simulink model "syste_analysis_i"  (R2024a)
settings: Solver=FixedStepAuto  StartTime=0.0  StopTime=10  FixedStep=0.01  RelTol=1e-3
undefined symbols (not defined in the file or in its folder): A_stable, B_num
settings Model: Creator=phili  LastModifiedBy=phili

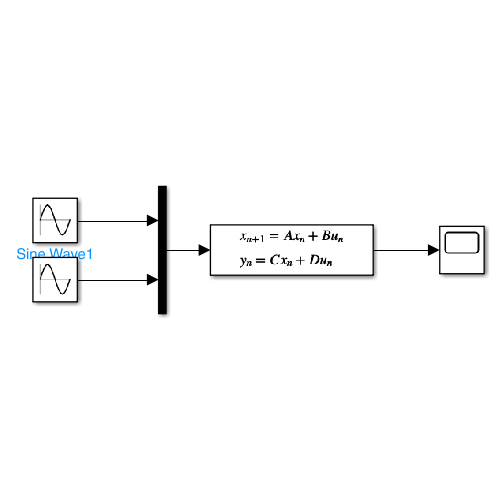
[thumbnail: Simulink's stored preview of the top-level diagram]
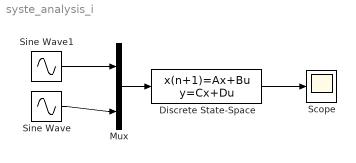
== system syste_analysis_i ==
  Discrete State-Space : DiscreteStateSpace  A=A_stable  B=B_num  C=eye(4)  D=zeros(4,2)  InitialCondition=[1,-1,2,4]  SampleTime=-1
  Mux : Mux  Inputs=2
  Scope : Scope
  Sine Wave : Sin  Frequency=20  SampleTime=0
  Sine Wave1 : Sin  Frequency=50  SampleTime=0
  wires:
  Discrete State-Space/1 -> Scope/1
  Sine Wave/1 -> Mux/2
  Mux/1 -> Discrete State-Space/1
  Sine Wave1/1 -> Mux/1
